simulink library "sharedController"  (R2020a)
settings: Solver=VariableStepAuto  StartTime=0.0  StopTime=10.0  RelTol=1e-3
undefined symbols (not defined in the file or in its folder): env, FLIGHTCONTROLLER, fltCtrl, share, vhcl
libraries: pathFollowingControllerExp_cl x1, periodicCtrlExpAllocate x1
settings Model: Creator=adabney  LastModifiedBy=adabney

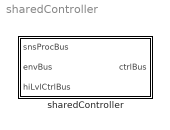
== system sharedController ==
  sharedController : Subsystem  mask{vhcl=vhcl, env=env, fltCtrl=fltCtrl}
      mask prompts: vhcl "Vehicle Model"; env "Environment Model"; fltCtrl "Flight Controller"

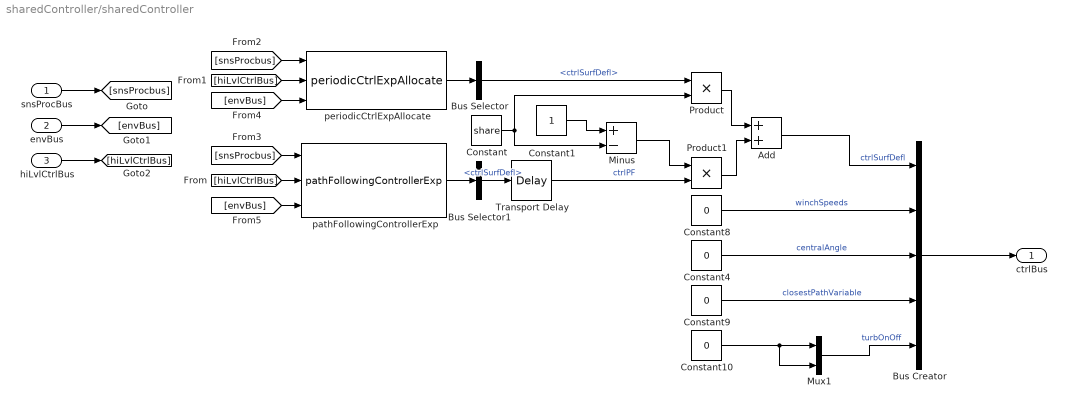
== system sharedController/sharedController ==
  snsProcBus : Inport  OutDataTypeStr=Bus: sensorsProcessingBus
  envBus : Inport  Port=2  OutDataTypeStr=Bus: envBus
  hiLvlCtrlBus : Inport  Port=3  OutDataTypeStr=Bus: hiLvlCtrlBus
  Add : Sum
  Bus Creator : BusCreator  Inputs=5  OutDataTypeStr=Bus: fltCtrlBus
      settings: InheritFromInputs=off
  Bus Selector : BusSelector  OutputSignals=ctrlSurfDefl
  Bus Selector1 : BusSelector  OutputSignals=ctrlSurfDefl
  Constant : Constant  Value=share
  Constant1 : Constant
  Constant{4,8..10} (4 alike) : Constant  Value=0
  Minus : Sum  Inputs=+-
  Mux1 : Mux  Inputs=2
  Product : Product
  Product1 : Product
  Transport Delay : TransportDelay  DelayTime=.03
  pathFollowingControllerExp : pathFollowingControllerExp_cl/pathFollowingControllerExp  VariantControl=strcmpi(FLIGHTCONTROLLER,'pathFollowingControllerExp')  initPosForInitSStar=vhcl.initPosVecGnd.Value  fluidDensity=env.water.density.Value  pathCtrl=fltCtrl  aeroStruct=vhcl.struct('OCT.aeroSurf')  thrAttach=vhcl.rBridle_LE.Value  vhcl=vhcl
  periodicCtrlExpAllocate : periodicCtrlExpAllocate/periodicCtrlExpAllocate  VariantControl=strcmpi(FLIGHTCONTROLLER,'periodicCtrlExpAllocate')  fltCtrl=fltCtrl
      link override Transport Delay: DelayTime=.03
  ctrlBus : Outport  OutDataTypeStr=Bus: fltCtrlBus  VectorParamsAs1DForOutWhenUnconnected=off
  wires:
  [hiLvlCtrlBus] -> periodicCtrlExpAllocate/2
  [snsProcbus] -> periodicCtrlExpAllocate/1
  Mux1/1 -> Bus Creator/5  "turbOnOff"
  envBus/1 -> [envBus]
  Constant4/1 -> Bus Creator/3  "centralAngle"
  Constant9/1 -> Bus Creator/4  "closestPathVariable"
  Bus Selector/1 -> Product/1  "<ctrlSurfDefl>"
  Constant10/1 -> Mux1/2, Mux1/1
  Transport Delay/1 -> Product1/2  "ctrlPF"
  Constant8/1 -> Bus Creator/2  "winchSpeeds"
  Constant/1 -> Minus/2, Product/2
  [envBus] -> periodicCtrlExpAllocate/3
  [hiLvlCtrlBus] -> pathFollowingControllerExp/2
  periodicCtrlExpAllocate/1 -> Bus Selector/1
  Product1/1 -> Add/2
  Bus Creator/1 -> ctrlBus/1
  snsProcBus/1 -> [snsProcbus]
  pathFollowingControllerExp/1 -> Bus Selector1/1
  Constant1/1 -> Minus/1
  Bus Selector1/1 -> Transport Delay/1  "<ctrlSurfDefl>"
  [snsProcbus] -> pathFollowingControllerExp/1
  [envBus] -> pathFollowingControllerExp/3
  hiLvlCtrlBus/1 -> [hiLvlCtrlBus]
  Minus/1 -> Product1/1
  Product/1 -> Add/1
  Add/1 -> Bus Creator/1  "ctrlSurfDefl"
